simulink model "Iek2"  (Simulink 8.7)
settings: Solver=FixedStepDiscrete  StartTime=0.0  StopTime=10000000.0  RelTol=1e-3
settings Model: Creator=scaife  LastModifiedBy=hamza  ExtModeAutoUpdateStatusClock=off
settings DataIOCC: SignalLoggingSaveFormat=ModelDataLogs  SignalLoggingName=sigsOut
settings DebuggingCC: SaveWithParameterizedLinksMsg=none  SignalResolutionControl=TryResolveAllWithWarning  MultiTaskDSMMsg=warning  MultiTaskCondExecSysMsg=none
settings HardwareCC: TargetUnknown=on
settings SFSimCC: SimParseCustomCode=off
settings GRTTargetCC: GeneratePreprocessorConditionals=Use local settings  CombineOutputUpdateFcns=off  GRTInterface=on

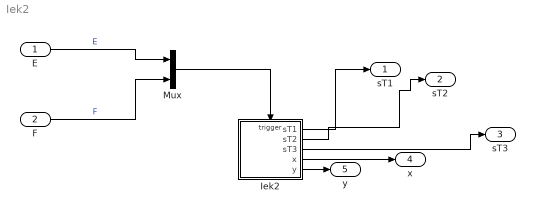
== system Iek2 ==
  E : Inport
  F : Inport  Port=2
  Iek2 : Stateflow chart  TreatAsAtomicUnit=on
  Mux : Mux  Inputs=2
  sT1 : Outport
  sT2 : Outport  Port=2
  sT3 : Outport  Port=3
  x : Outport  Port=4
  y : Outport  Port=5
  wires:
  Mux/1 -> Iek2/Trigger
  F/1 -> Mux/2  "F"
  E/1 -> Mux/1  "E"
  Iek2/1(sT1) -> sT1/1
  Iek2/2(sT2) -> sT2/1
  Iek2/3(sT3) -> sT3/1
  Iek2/4(x) -> x/1
  Iek2/5(y) -> y/1

== stateflow chart Iek2 ==
  state T1 [parallel]
    settings: executionOrder=1
    state B
      en: sT1=2
    state A
      en: sT1=1
    (default) -> A
    B -> A : E{x++}
    A -> B : E{x++}
  state T2 [parallel]
    settings: executionOrder=2
    state C/
      en: y++;
      sT2=1
    state D/
      en: y++;
      sT2=2
    (default) -> C
    D -> C : F
    C -> D : F
  state T3 [parallel]
    settings: executionOrder=3
    state a
      en: sT3=1
    state c
      en: sT3=3
    state b
      en: sT3=2
    state d
      en: sT3=4
    (default) -> a
    a -> c : change(x)
    b -> c [order 2] : change(x)
    b -> a [order 1] : change(y)
    c -> b [order 2] : change(y)
    c -> d [order 1] : change(x)
    d -> b : change(y)
  data: sT1 output int8; sT2 output int8; sT3 output int8; x output int8; y output int8
  events: E input EITHER_EDGE_EVENT; F input EITHER_EDGE_EVENT
